simulink model "Demo"  (R2019a)
settings: Solver=VariableStepAuto  StartTime=0.0  StopTime=5  FixedStep=10e-6  RelTol=1e-3
StopFcn:
  | run PlotResults.m
settings Model: Creator=visha  LastModifiedBy=visha
settings SolverCC: AlgebraicLoopSolver=LineSearch

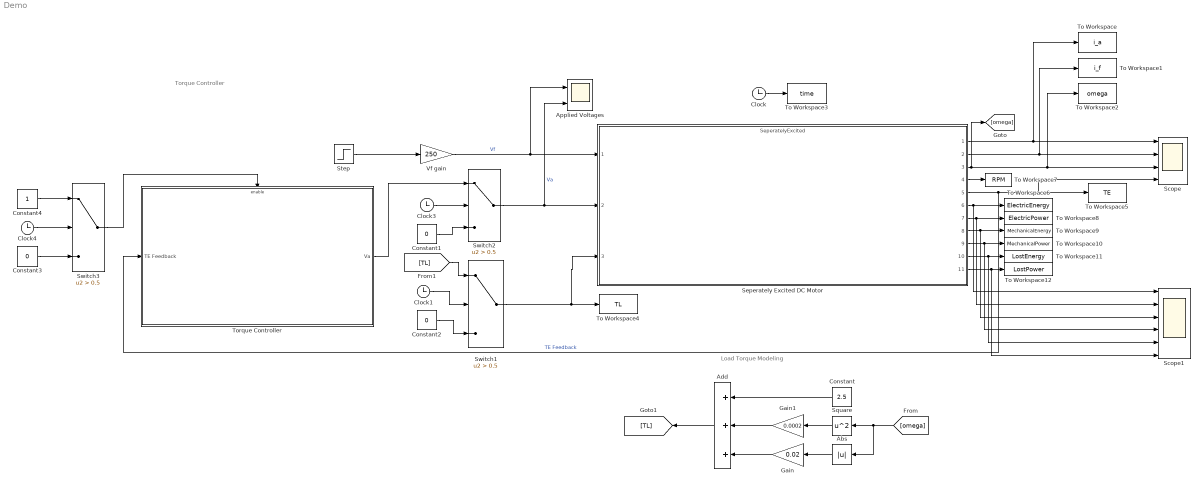
== system Demo ==
  note: Load Torque Modeling
  note: Torque Controller
  Abs : Abs
  Add : Sum  Inputs=+++
  "Applied Voltages " : Scope  NumInputPorts=2
  Clock{,1,3..4} (4 alike) : Clock
  Constant : Constant  Value=2.5
  Constant1 : Constant  Value=0
  Constant2 : Constant  Value=0
  Constant3 : Constant  Value=0
  Constant4 : Constant
  Gain : Gain  Gain=0.02
  Gain1 : Gain  Gain=0.0002
  Scope : Scope  NumInputPorts=4
  Scope1 : Scope  NumInputPorts=6
  "Seperately Excited DC Motor " : ModelReference  ModelNameDialog=SeperatelyExcited.slx  SimulationMode=Normal  ModelReferenceVersion=1.27
  Square : Math  Operator=square  SaturateOnIntegerOverflow=on
  Step : Step  Time=0  SampleTime=0
  Switch1 : Switch  Criteria=u2 > Threshold  Threshold=0.5
  Switch2 : Switch  Criteria=u2 > Threshold  Threshold=0.5
  Switch3 : Switch  Criteria=u2 > Threshold  Threshold=0.5
  To Workspace : ToWorkspace  VariableName=i_a  SaveFormat=Timeseries  SampleTime=-1
  To Workspace1 : ToWorkspace  VariableName=i_f  SaveFormat=Timeseries  SampleTime=-1
  To Workspace10 : ToWorkspace  VariableName=MechanicalPower  SaveFormat=Timeseries  SampleTime=-1
  To Workspace11 : ToWorkspace  VariableName=LostEnergy  SaveFormat=Timeseries  SampleTime=-1
  To Workspace12 : ToWorkspace  VariableName=LostPower  SaveFormat=Timeseries  SampleTime=-1
  To Workspace2 : ToWorkspace  VariableName=omega  SaveFormat=Timeseries  SampleTime=-1
  To Workspace3 : ToWorkspace  VariableName=time  SaveFormat=Timeseries  SampleTime=-1
  To Workspace4 : ToWorkspace  VariableName=TL  SaveFormat=Timeseries  SampleTime=-1
  To Workspace5 : ToWorkspace  VariableName=TE  SaveFormat=Timeseries  SampleTime=-1
  To Workspace6 : ToWorkspace  VariableName=ElectricEnergy  SaveFormat=Timeseries  SampleTime=-1
  To Workspace7 : ToWorkspace  VariableName=RPM  SaveFormat=Timeseries  SampleTime=-1
  To Workspace8 : ToWorkspace  VariableName=ElectricPower  SaveFormat=Timeseries  SampleTime=-1
  To Workspace9 : ToWorkspace  VariableName=MechanicalEnergy  SaveFormat=Timeseries  SampleTime=-1
  Torque Controller : Subsystem
  Vf gain : Gain  Gain=250
  wires:
  Square/1 -> Gain1/1
  Abs/1 -> Gain/1
  Gain/1 -> Add/3
  Gain1/1 -> Add/2
  Constant/1 -> Add/1
  [omega] -> Abs/1, Square/1
  "Seperately Excited DC Motor "/3 -> Scope/3, To Workspace2/1, [omega]
  Add/1 -> [TL]
  "Seperately Excited DC Motor "/1 -> Scope/1, To Workspace/1
  "Seperately Excited DC Motor "/2 -> Scope/2, To Workspace1/1
  Clock/1 -> To Workspace3/1
  "Seperately Excited DC Motor "/5 -> Torque Controller/1(TE Feedback), Scope/4, To Workspace5/1  "TE Feedback"
  "Seperately Excited DC Motor "/7 -> Scope1/2, To Workspace8/1
  "Seperately Excited DC Motor "/8 -> Scope1/3, To Workspace9/1
  "Seperately Excited DC Motor "/6 -> Scope1/1, To Workspace6/1
  "Seperately Excited DC Motor "/9 -> Scope1/4, To Workspace10/1
  "Seperately Excited DC Motor "/10 -> Scope1/5, To Workspace11/1
  "Seperately Excited DC Motor "/11 -> Scope1/6, To Workspace12/1
  "Seperately Excited DC Motor "/4 -> To Workspace7/1
  Clock1/1 -> Switch1/2
  [TL] -> Switch1/1
  Constant2/1 -> Switch1/3
  Switch1/1 -> "Seperately Excited DC Motor "/3, To Workspace4/1
  Step/1 -> Vf gain/1
  Vf gain/1 -> "Applied Voltages "/1, "Seperately Excited DC Motor "/1  "Vf"
  Torque Controller/1(Va) -> Switch2/1
  Clock3/1 -> Switch2/2
  Constant1/1 -> Switch2/3
  Switch2/1 -> "Seperately Excited DC Motor "/2, "Applied Voltages "/2  "Va"
  Constant3/1 -> Switch3/3
  Clock4/1 -> Switch3/2
  Constant4/1 -> Switch3/1
  Switch3/1 -> Torque Controller/Enable

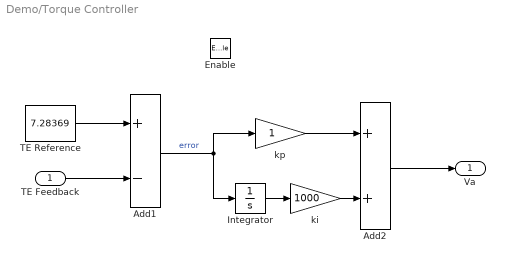
== system Demo/Torque Controller ==
  TE Feedback : Inport
  Enable : EnablePort
  Add1 : Sum  Inputs=+-
  Add2 : Sum
  Integrator : Integrator
  TE Reference : Constant  Value=7.28369
  ki : Gain  Gain=1000
  kp : Gain
  Va : Outport
  wires:
  ki/1 -> Add2/2
  Add2/1 -> Va/1
  Add1/1 -> Integrator/1, kp/1  "error"
  TE Reference/1 -> Add1/1
  kp/1 -> Add2/1
  Integrator/1 -> ki/1
  TE Feedback/1 -> Add1/2
